simulink model "BlockDiagram_Detailed_Fluids"  (R2025b)
settings: Solver=VariableStepAuto  StartTime=0.0  StopTime=10.0  RelTol=1e-3
values from neighbouring files (symbols this model uses):
  CdA_max_valve_ox = mdot_ox_nom / sqrt(2 * rho_ox * DeltaP_valve_ox)    [calculate_desired_Cv_range.m]
  P_amb = 101325    [init_engine_params.m]
  P_tank_f = 3242543.676    [init_engine_params.m]
  P_tank_ox = 3260949.847    [init_engine_params.m]
  rho_f = 789    [init_engine_params.m]
  rho_ox = 988.82    [init_engine_params.m]
  V_c = 2.5335373958699e-4    (= 0.000253353739587)    [init_engine_params.m]
undefined symbols (not defined in the file or in its folder): a_liq_f, a_liq_ox, CdA_inj_f, CdA_inj_ox, V_plenum_f, V_plenum_ox
settings Model: Creator=gruby  LastModifiedBy=gruby

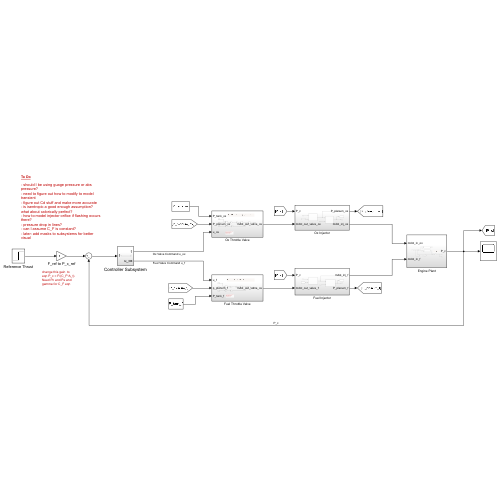
[thumbnail: Simulink's stored preview of the top-level diagram]
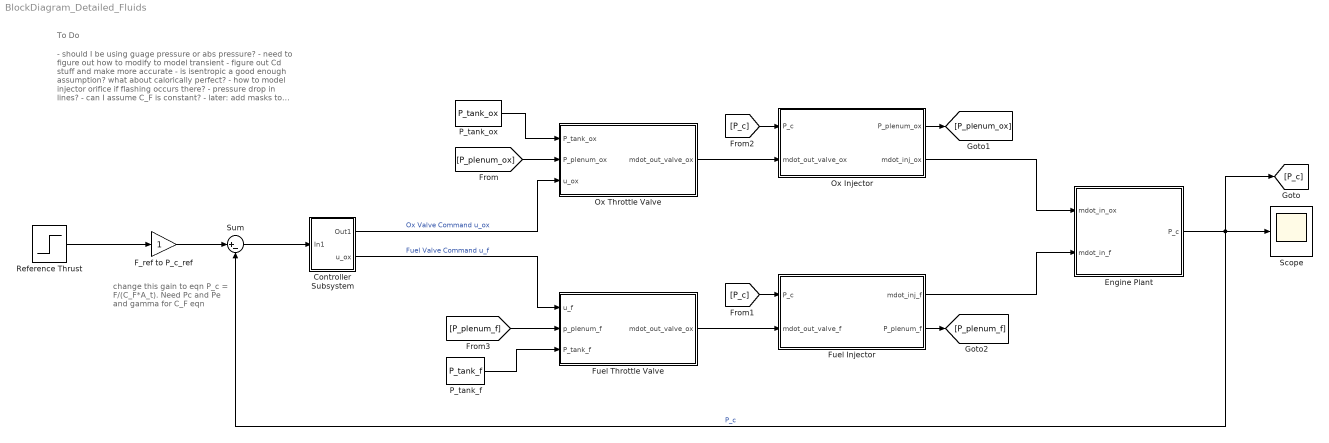
== system BlockDiagram_Detailed_Fluids ==
  note: To Do
  note: - should I be using guage pressure or abs pressure?
      | - need to figure out how to modify to model transient
      | - figure out Cd stuff and make more accurate
      | - is isentropic a good enough assumption? what about calorically perfect?
      | - how to model injector orifice if flashing occurs there?
      | - pressure drop in lines?
      | - can I assume C_F is constant?
      | - later: add masks to subsystems for better visual
  note: change this gain to eqn P_c = F/(C_F*A_t). Need Pc and Pe and gamma for C_F eqn
  Controller Subsystem : Subsystem
  Engine Plant : Subsystem
  F_ref to P_c_ref : Gain
  Fuel Injector : Subsystem
  Fuel Throttle Valve : Subsystem
  Ox Injector : Subsystem
  Ox Throttle Valve : Subsystem
  P_tank_f : Constant  Value=P_tank_f
  P_tank_ox : Constant  Value=P_tank_ox
  Reference Thrust : Step  SampleTime=0
  Scope : Scope
      settings: ActiveDisplayYMinimum=-1.8374784378622904  ActiveDisplayYMaximum=16.537497604206919
  Sum : Sum  Inputs=|+-
  wires:
  Sum/1 -> Controller Subsystem/1(In1)
  F_ref to P_c_ref/1 -> Sum/1
  Reference Thrust/1 -> F_ref to P_c_ref/1
  Engine Plant/1(P_c) -> Scope/1, [P_c], Sum/2  "P_c"
  [P_c] -> Ox Injector/1(P_c)
  Controller Subsystem/1(Out1) -> Ox Throttle Valve/3(u_ox)  "Ox Valve Command u_ox"
  Controller Subsystem/2(u_ox) -> Fuel Throttle Valve/1(u_f)  "Fuel Valve Command u_f"
  P_tank_ox/1 -> Ox Throttle Valve/1(P_tank_ox)
  Ox Throttle Valve/1(mdot_out_valve_ox) -> Ox Injector/2(mdot_out_valve_ox)
  P_tank_f/1 -> Fuel Throttle Valve/3(P_tank_f)
  [P_c] -> Fuel Injector/1(P_c)
  Fuel Throttle Valve/1(mdot_out_valve_ox) -> Fuel Injector/2(mdot_out_valve_f)
  Ox Injector/2(mdot_inj_ox) -> Engine Plant/1(mdot_in_ox)
  Fuel Injector/1(mdot_inj_f) -> Engine Plant/2(mdot_in_f)
  Ox Injector/1(P_plenum_ox) -> [P_plenum_ox]
  [P_plenum_ox] -> Ox Throttle Valve/2(P_plenum_ox)
  Fuel Injector/2(P_plenum_f) -> [P_plenum_f]
  [P_plenum_f] -> Fuel Throttle Valve/2(p_plenum_f)

== system BlockDiagram_Detailed_Fluids/Controller Subsystem ==
  In1 : Inport
  Out1 : Outport
  u_ox : Outport  Port=2
  wires:
  In1/1 -> u_ox/1, Out1/1

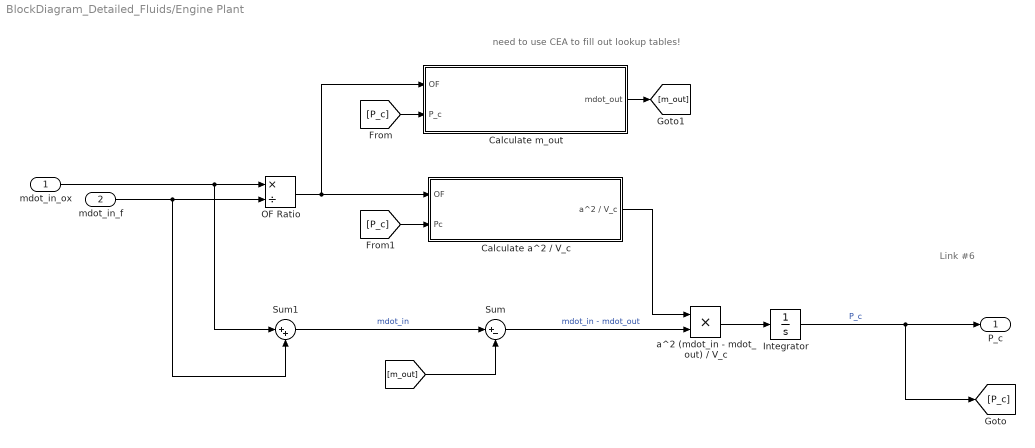
== system BlockDiagram_Detailed_Fluids/Engine Plant ==
  note: Link #6
  note: need to use CEA to fill out lookup tables!
  mdot_in_ox : Inport
  mdot_in_f : Inport  Port=2
  Calculate a^2 / V_c : Subsystem
  Calculate m_out : Subsystem
  Integrator : Integrator  InitialCondition=P_amb
  OF Ratio : Product  Inputs=*/
  Sum : Sum  Inputs=|+-
  Sum1 : Sum  Inputs=|++
  "a^2 (mdot_in - mdot_out) / V_c " : Product
  P_c : Outport
  wires:
  mdot_in_f/1 -> Sum1/2, OF Ratio/2
  mdot_in_ox/1 -> Sum1/1, OF Ratio/1
  Sum/1 -> "a^2 (mdot_in - mdot_out) / V_c "/2  "mdot_in - mdot_out"
  Integrator/1 -> P_c/1, [P_c]  "P_c"
  OF Ratio/1 -> Calculate m_out/1(OF), Calculate a^2 / V_c/1(OF)
  Sum1/1 -> Sum/1  "mdot_in"
  "a^2 (mdot_in - mdot_out) / V_c "/1 -> Integrator/1
  [P_c] -> Calculate m_out/2(P_c)
  [P_c] -> Calculate a^2 / V_c/2(Pc)
  Calculate a^2 / V_c/1(a^2 / V_c) -> "a^2 (mdot_in - mdot_out) / V_c "/1
  Calculate m_out/1(mdot_out) -> [m_out]
  [m_out] -> Sum/2

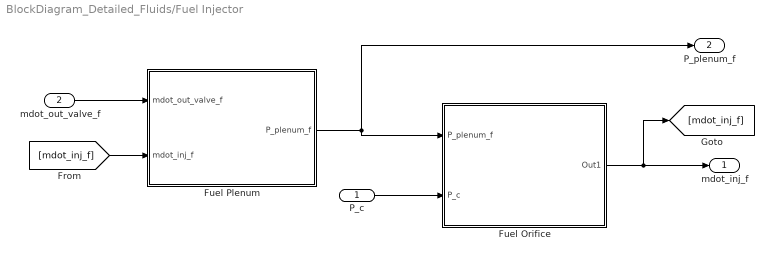
== system BlockDiagram_Detailed_Fluids/Fuel Injector ==
  P_c : Inport
  mdot_out_valve_f : Inport  Port=2
  Fuel Orifice : Subsystem
  Fuel Plenum : Subsystem
  mdot_inj_f : Outport
  P_plenum_f : Outport  Port=2
  wires:
  mdot_out_valve_f/1 -> Fuel Plenum/1(mdot_out_valve_f)
  [mdot_inj_f] -> Fuel Plenum/2(mdot_inj_f)
  Fuel Orifice/1(Out1) -> [mdot_inj_f], mdot_inj_f/1
  Fuel Plenum/1(P_plenum_f) -> P_plenum_f/1, Fuel Orifice/1(P_plenum_f)
  P_c/1 -> Fuel Orifice/2(P_c)

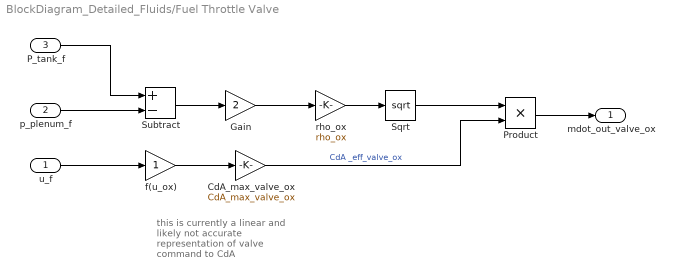
== system BlockDiagram_Detailed_Fluids/Fuel Throttle Valve ==
  note: this is currently a linear and likely not accurate representation of valve command to CdA
  u_f : Inport
  p_plenum_f : Inport  Port=2
  P_tank_f : Inport  Port=3
  CdA_max_valve_ox : Gain  Gain=CdA_max_valve_ox
  Gain : Gain  Gain=2
  Product : Product
  Sqrt : Sqrt
  Subtract : Sum  Inputs=+-
  f(u_ox) : Gain
  rho_ox : Gain  Gain=rho_ox
  mdot_out_valve_ox : Outport
  wires:
  f(u_ox)/1 -> CdA_max_valve_ox/1
  u_f/1 -> f(u_ox)/1
  CdA_max_valve_ox/1 -> Product/2  "CdA _eff_valve_ox"
  P_tank_f/1 -> Subtract/1
  Subtract/1 -> Gain/1
  Gain/1 -> rho_ox/1
  rho_ox/1 -> Sqrt/1
  Sqrt/1 -> Product/1
  Product/1 -> mdot_out_valve_ox/1
  p_plenum_f/1 -> Subtract/2

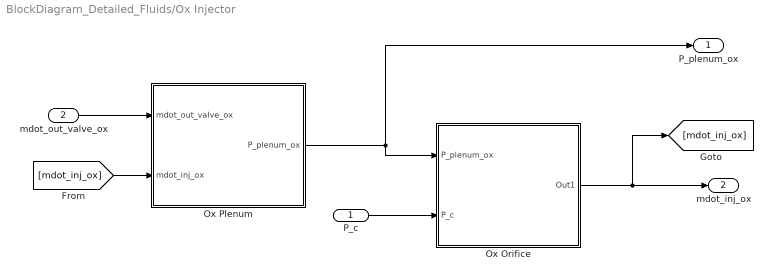
== system BlockDiagram_Detailed_Fluids/Ox Injector ==
  P_c : Inport
  mdot_out_valve_ox : Inport  Port=2
  Ox Orifice : Subsystem
  Ox Plenum : Subsystem
  P_plenum_ox : Outport
  mdot_inj_ox : Outport  Port=2
  wires:
  mdot_out_valve_ox/1 -> Ox Plenum/1(mdot_out_valve_ox)
  [mdot_inj_ox] -> Ox Plenum/2(mdot_inj_ox)
  Ox Orifice/1(Out1) -> [mdot_inj_ox], mdot_inj_ox/1
  Ox Plenum/1(P_plenum_ox) -> P_plenum_ox/1, Ox Orifice/1(P_plenum_ox)
  P_c/1 -> Ox Orifice/2(P_c)

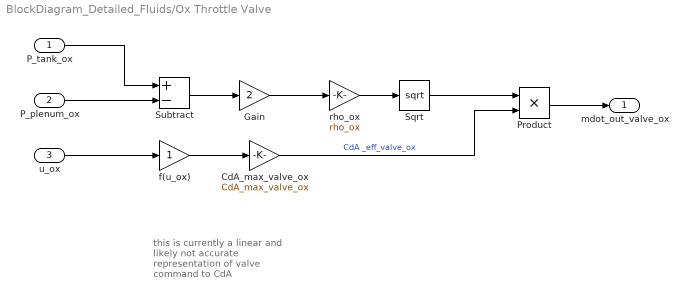
== system BlockDiagram_Detailed_Fluids/Ox Throttle Valve ==
  note: this is currently a linear and likely not accurate representation of valve command to CdA
  P_tank_ox : Inport
  P_plenum_ox : Inport  Port=2
  u_ox : Inport  Port=3
  CdA_max_valve_ox : Gain  Gain=CdA_max_valve_ox
  Gain : Gain  Gain=2
  Product : Product
  Sqrt : Sqrt
  Subtract : Sum  Inputs=+-
  f(u_ox) : Gain
  rho_ox : Gain  Gain=rho_ox
  mdot_out_valve_ox : Outport
  wires:
  f(u_ox)/1 -> CdA_max_valve_ox/1
  u_ox/1 -> f(u_ox)/1
  CdA_max_valve_ox/1 -> Product/2  "CdA _eff_valve_ox"
  P_tank_ox/1 -> Subtract/1
  P_plenum_ox/1 -> Subtract/2
  Subtract/1 -> Gain/1
  Gain/1 -> rho_ox/1
  rho_ox/1 -> Sqrt/1
  Sqrt/1 -> Product/1
  Product/1 -> mdot_out_valve_ox/1

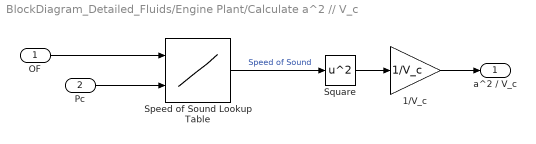
== system BlockDiagram_Detailed_Fluids/Engine Plant/Calculate a^2 // V_c ==
  OF : Inport
  Pc : Inport  Port=2
  1/V_c : Gain  Gain=1/V_c
  Speed of Sound Lookup Table : Lookup_n-D  BreakpointsForDimension1=[1:3]  BreakpointsForDimension2=[1:3]  InternalRulePriority=Speed  RndMeth=Simplest
      settings: InputPortMap=u0,u1
  Square : Math  Operator=square
  a^2 / V_c : Outport
  wires:
  Speed of Sound Lookup Table/1 -> Square/1  "Speed of Sound"
  OF/1 -> Speed of Sound Lookup Table/1
  Square/1 -> 1/V_c/1
  Pc/1 -> Speed of Sound Lookup Table/2
  1/V_c/1 -> a^2 / V_c/1

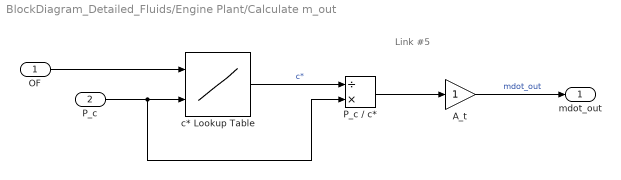
== system BlockDiagram_Detailed_Fluids/Engine Plant/Calculate m_out ==
  note: Link #5
  OF : Inport
  P_c : Inport  Port=2
  A_t : Gain
  P_c / c* : Product  Inputs=/*
  c* Lookup Table : Lookup_n-D  BreakpointsForDimension1=[1:3]  BreakpointsForDimension2=[1:3]  InternalRulePriority=Speed  RndMeth=Simplest
      settings: InputPortMap=u0,u1
  mdot_out : Outport
  wires:
  c* Lookup Table/1 -> P_c / c*/1  "c*"
  P_c / c*/1 -> A_t/1
  OF/1 -> c* Lookup Table/1
  A_t/1 -> mdot_out/1  "mdot_out"
  P_c/1 -> P_c / c*/2, c* Lookup Table/2

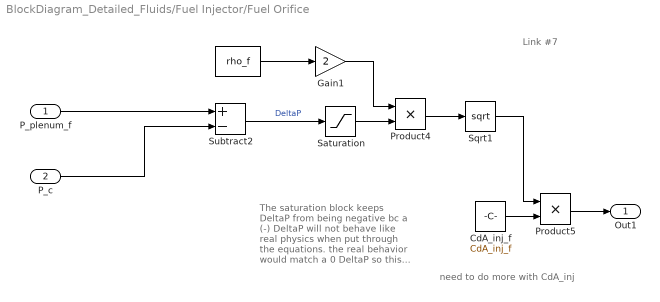
== system BlockDiagram_Detailed_Fluids/Fuel Injector/Fuel Orifice ==
  note: need to do more with CdA_inj
  note: Link #7
  note: The saturation block keeps DeltaP from being negative bc a (-) DeltaP will not behave like real physics when put through the equations. the real behavior would match a 0 DeltaP so this makes a lower lim of 0.
  P_plenum_f : Inport
  P_c : Inport  Port=2
  "   " : Constant  Value=rho_f
  CdA_inj_f : Constant  Value=CdA_inj_f
  Gain1 : Gain  Gain=2
  Product4 : Product
  Product5 : Product
  Saturation : Saturate  LowerLimit=0
  Sqrt1 : Sqrt
  Subtract2 : Sum  Inputs=+-
  Out1 : Outport
  wires:
  Saturation/1 -> Product4/2
  Gain1/1 -> Product4/1
  Product5/1 -> Out1/1
  Product4/1 -> Sqrt1/1
  CdA_inj_f/1 -> Product5/2
  Sqrt1/1 -> Product5/1
  Subtract2/1 -> Saturation/1  "DeltaP"
  "   "/1 -> Gain1/1
  P_c/1 -> Subtract2/2
  P_plenum_f/1 -> Subtract2/1

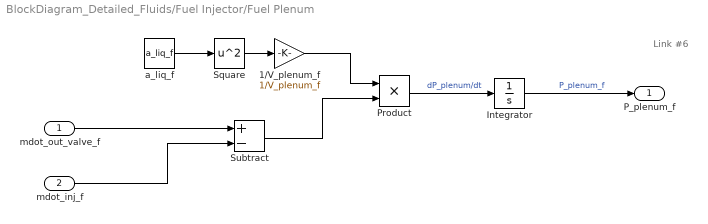
== system BlockDiagram_Detailed_Fluids/Fuel Injector/Fuel Plenum ==
  note: Link #6
  mdot_out_valve_f : Inport
  mdot_inj_f : Inport  Port=2
  1/V_plenum_f : Gain  Gain=1/V_plenum_f
  Integrator : Integrator
  Product : Product
  Square : Math  Operator=square
  Subtract : Sum  Inputs=+-
  a_liq_f : Constant  Value=a_liq_f
  P_plenum_f : Outport
  wires:
  Integrator/1 -> P_plenum_f/1  "P_plenum_f"
  1/V_plenum_f/1 -> Product/1
  mdot_inj_f/1 -> Subtract/2
  mdot_out_valve_f/1 -> Subtract/1
  Square/1 -> 1/V_plenum_f/1
  Subtract/1 -> Product/2
  a_liq_f/1 -> Square/1
  Product/1 -> Integrator/1  "dP_plenum/dt"

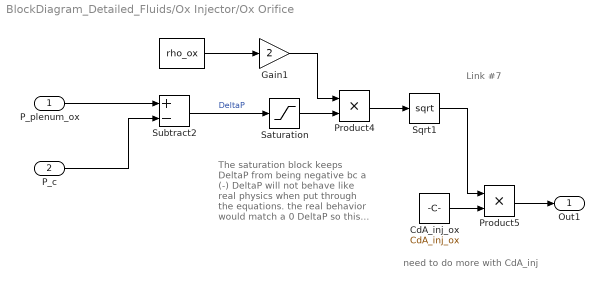
== system BlockDiagram_Detailed_Fluids/Ox Injector/Ox Orifice ==
  note: Link #7
  note: The saturation block keeps DeltaP from being negative bc a (-) DeltaP will not behave like real physics when put through the equations. the real behavior would match a 0 DeltaP so this makes a lower lim of 0.
  note: need to do more with CdA_inj
  P_plenum_ox : Inport
  P_c : Inport  Port=2
  "   " : Constant  Value=rho_ox
  CdA_inj_ox : Constant  Value=CdA_inj_ox
  Gain1 : Gain  Gain=2
  Product4 : Product
  Product5 : Product
  Saturation : Saturate  LowerLimit=0
  Sqrt1 : Sqrt
  Subtract2 : Sum  Inputs=+-
  Out1 : Outport
  wires:
  Saturation/1 -> Product4/2
  Gain1/1 -> Product4/1
  Product5/1 -> Out1/1
  Product4/1 -> Sqrt1/1
  CdA_inj_ox/1 -> Product5/2
  Sqrt1/1 -> Product5/1
  Subtract2/1 -> Saturation/1  "DeltaP"
  "   "/1 -> Gain1/1
  P_c/1 -> Subtract2/2
  P_plenum_ox/1 -> Subtract2/1

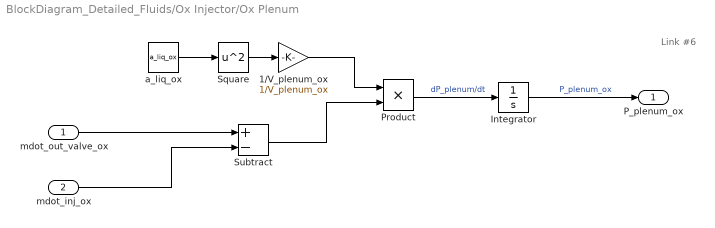
== system BlockDiagram_Detailed_Fluids/Ox Injector/Ox Plenum ==
  note: Link #6
  mdot_out_valve_ox : Inport
  mdot_inj_ox : Inport  Port=2
  1/V_plenum_ox : Gain  Gain=1/V_plenum_ox
  Integrator : Integrator
  Product : Product
  Square : Math  Operator=square
  Subtract : Sum  Inputs=+-
  a_liq_ox : Constant  Value=a_liq_ox
  P_plenum_ox : Outport
  wires:
  Integrator/1 -> P_plenum_ox/1  "P_plenum_ox"
  1/V_plenum_ox/1 -> Product/1
  mdot_inj_ox/1 -> Subtract/2
  mdot_out_valve_ox/1 -> Subtract/1
  Square/1 -> 1/V_plenum_ox/1
  Subtract/1 -> Product/2
  a_liq_ox/1 -> Square/1
  Product/1 -> Integrator/1  "dP_plenum/dt"
